simulink model "genericjosephtest"  (Simulink 10.3)
settings: Solver=ode45  StartTime=0.0  StopTime=inf  RelTol=1e-3  EnableMultiTasking=on
values from neighbouring files (symbols this model uses):
  ku = (Lr*m)/(Cyf*(Lf+Lr)) - (Lf*m)/(Cyr*(Lf+Lr))    (= -0.00270204285714)    [makePlants.m]
  Lf = 0.918    [makeBikeModel.m]    (also in makePlants.m)
  Lr = 0.612    [makeBikeModel.m]    (also in makePlants.m)
undefined symbols (not defined in the file or in its folder): Gains
libraries: CarMaker4SL x24, slctrlblks x2, pid_lib x2, simulink x1
(part 3 of 3)

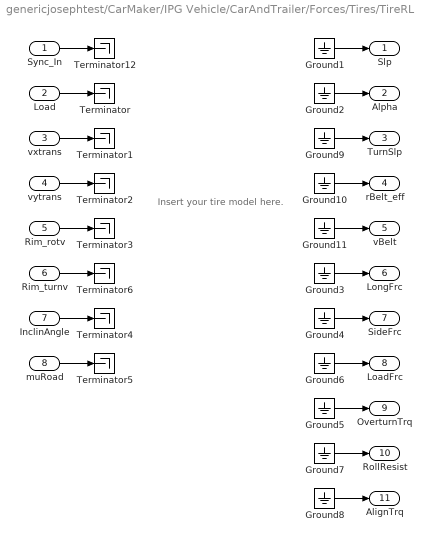
== system genericjosephtest/CarMaker/IPG Vehicle/CarAndTrailer/Forces/Tires/TireRL ==
  note: Insert your tire model here.
  Sync_In : Inport
  Load : Inport  Port=2
  vxtrans : Inport  Port=3
  vytrans : Inport  Port=4
  Rim_rotv : Inport  Port=5
  Rim_turnv : Inport  Port=6
  InclinAngle : Inport  Port=7
  muRoad : Inport  Port=8
  Ground{1..11} (11 alike) : Ground
  Terminator{,1..6,12} (8 alike) : Terminator
  Slp : Outport  VectorParamsAs1DForOutWhenUnconnected=off
  Alpha : Outport  Port=2  VectorParamsAs1DForOutWhenUnconnected=off
  TurnSlp : Outport  Port=3  VectorParamsAs1DForOutWhenUnconnected=off
  rBelt_eff : Outport  Port=4  VectorParamsAs1DForOutWhenUnconnected=off
  vBelt : Outport  Port=5  VectorParamsAs1DForOutWhenUnconnected=off
  LongFrc : Outport  Port=6  VectorParamsAs1DForOutWhenUnconnected=off
  SideFrc : Outport  Port=7  VectorParamsAs1DForOutWhenUnconnected=off
  LoadFrc : Outport  Port=8  VectorParamsAs1DForOutWhenUnconnected=off
  OverturnTrq : Outport  Port=9  VectorParamsAs1DForOutWhenUnconnected=off
  RollResist : Outport  Port=10  VectorParamsAs1DForOutWhenUnconnected=off
  AlignTrq : Outport  Port=11  VectorParamsAs1DForOutWhenUnconnected=off
  wires:
  Ground11/1 -> vBelt/1
  Ground10/1 -> rBelt_eff/1
  Ground9/1 -> TurnSlp/1
  Rim_turnv/1 -> Terminator6/1
  Sync_In/1 -> Terminator12/1
  Ground2/1 -> Alpha/1
  Ground3/1 -> LongFrc/1
  Ground4/1 -> SideFrc/1
  Ground5/1 -> OverturnTrq/1
  vxtrans/1 -> Terminator1/1
  vytrans/1 -> Terminator2/1
  Rim_rotv/1 -> Terminator3/1
  InclinAngle/1 -> Terminator4/1
  muRoad/1 -> Terminator5/1
  Load/1 -> Terminator/1
  Ground1/1 -> Slp/1
  Ground6/1 -> LoadFrc/1
  Ground7/1 -> RollResist/1
  Ground8/1 -> AlignTrq/1

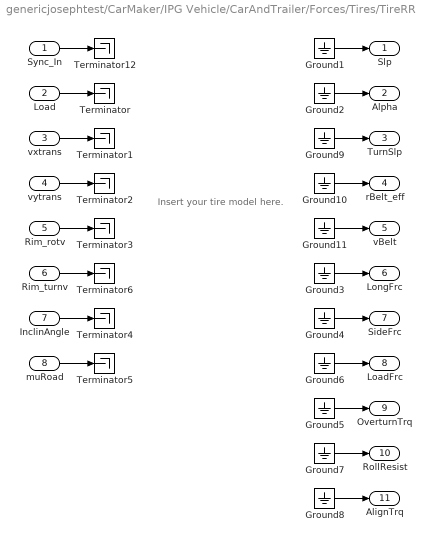
== system genericjosephtest/CarMaker/IPG Vehicle/CarAndTrailer/Forces/Tires/TireRR ==
  note: Insert your tire model here.
  Sync_In : Inport
  Load : Inport  Port=2
  vxtrans : Inport  Port=3
  vytrans : Inport  Port=4
  Rim_rotv : Inport  Port=5
  Rim_turnv : Inport  Port=6
  InclinAngle : Inport  Port=7
  muRoad : Inport  Port=8
  Ground{1..11} (11 alike) : Ground
  Terminator{,1..6,12} (8 alike) : Terminator
  Slp : Outport  VectorParamsAs1DForOutWhenUnconnected=off
  Alpha : Outport  Port=2  VectorParamsAs1DForOutWhenUnconnected=off
  TurnSlp : Outport  Port=3  VectorParamsAs1DForOutWhenUnconnected=off
  rBelt_eff : Outport  Port=4  VectorParamsAs1DForOutWhenUnconnected=off
  vBelt : Outport  Port=5  VectorParamsAs1DForOutWhenUnconnected=off
  LongFrc : Outport  Port=6  VectorParamsAs1DForOutWhenUnconnected=off
  SideFrc : Outport  Port=7  VectorParamsAs1DForOutWhenUnconnected=off
  LoadFrc : Outport  Port=8  VectorParamsAs1DForOutWhenUnconnected=off
  OverturnTrq : Outport  Port=9  VectorParamsAs1DForOutWhenUnconnected=off
  RollResist : Outport  Port=10  VectorParamsAs1DForOutWhenUnconnected=off
  AlignTrq : Outport  Port=11  VectorParamsAs1DForOutWhenUnconnected=off
  wires:
  Ground11/1 -> vBelt/1
  Ground10/1 -> rBelt_eff/1
  Ground9/1 -> TurnSlp/1
  Rim_turnv/1 -> Terminator6/1
  Sync_In/1 -> Terminator12/1
  Ground2/1 -> Alpha/1
  Ground3/1 -> LongFrc/1
  Ground4/1 -> SideFrc/1
  Ground5/1 -> OverturnTrq/1
  vxtrans/1 -> Terminator1/1
  vytrans/1 -> Terminator2/1
  Rim_rotv/1 -> Terminator3/1
  InclinAngle/1 -> Terminator4/1
  muRoad/1 -> Terminator5/1
  Load/1 -> Terminator/1
  Ground1/1 -> Slp/1
  Ground6/1 -> LoadFrc/1
  Ground7/1 -> RollResist/1
  Ground8/1 -> AlignTrq/1

== system genericjosephtest/CarMaker/IPG Vehicle/PowerTrain/MyPowerTrainXWD/Subsystem/Desired Yaw Rate Generator ==
  Linear Car Velocity : Inport
  steering angle : Inport  Port=2
  Add : Sum  Inputs=+++
  Constant : Constant  Value=0.8
  Constant1 : Constant  Value=ku
  Constant2 : Constant  Value=1.0
  Divide : Product  Inputs=*/
  Multiply : Product
  Multiply1 : Product
  Square : Math  Operator=square  SignedPower=on  SaturateOnIntegerOverflow=on
  Desired Yaw Rate : Outport  VectorParamsAs1DForOutWhenUnconnected=off
  wires:
  Constant1/1 -> Multiply/1
  steering angle/1 -> Multiply1/2
  Divide/1 -> Desired Yaw Rate/1
  Linear Car Velocity/1 -> Square/1, Multiply1/1
  Multiply/1 -> Add/1
  Multiply1/1 -> Divide/1
  Square/1 -> Multiply/2
  Constant/1 -> Add/2  "Lf - Distance between CG and front axel"
  Constant2/1 -> Add/3  "Lr - Distance between CG and rear axel"
  Add/1 -> Divide/2

== system genericjosephtest/CarMaker/IPG Vehicle/PowerTrain/MyPowerTrainXWD/Subsystem/Reference Yaw Rate Limiter ==
  note: Bind the reference yaw rate to the max possible yaw rate if the desired yaw rate is more than the max yaw rate possible
  note: Max Yaw Rate = tunability*mu*g/Vcg
  Vehicle Velocity : Inport
  Desired Yaw Rate : Inport  Port=2
  Add : Sum
  Constant : Constant  Value=2
  Constant1 : Constant  Value=0
  Divide : Product  Inputs=*/
  Divide1 : Product  Inputs=*/
  MATLAB Function : MATLAB Function  TreatAsAtomicUnit=on
  Multiply : Product
  Multiply1 : Product
  Read CM Dict : CarMaker4SL/Read CM Dict  xname=Car.muRoadRL  xsync=off
  Read CM Dict1 : CarMaker4SL/Read CM Dict  xname=Car.muRoadRR  xsync=off
  Saturation : Saturate  UpperLimit=10  LowerLimit=-10
  Switch : Switch  Criteria=u2 > Threshold  Threshold=1
  Tunability Factor : Constant
  g : Constant  Value=9.81
  Reference Yaw Rate : Outport  VectorParamsAs1DForOutWhenUnconnected=off
  wires:
  Desired Yaw Rate/1 -> Saturation/1
  MATLAB Function/1(ref_yaw) -> Reference Yaw Rate/1  "Reference Yaw Rate"
  Read CM Dict1/1 -> Add/2
  Read CM Dict/1 -> Add/1
  Add/1 -> Divide/1
  Constant/1 -> Divide/2
  Divide/1 -> Multiply/1  "mu (avg)"
  Multiply/1 -> Divide1/1
  Vehicle Velocity/1 -> Switch/2, Divide1/2
  g/1 -> Multiply/2
  Tunability Factor/1 -> Multiply1/2
  Multiply1/1 -> MATLAB Function/1(max_yaw)  "Max Yaw Rate"
  Divide1/1 -> Switch/1
  Constant1/1 -> Switch/3
  Switch/1 -> Multiply1/1
  Saturation/1 -> MATLAB Function/2(des_yaw)

== system genericjosephtest/CarMaker/IPG Vehicle/PowerTrain/MyPowerTrainXWD/Subsystem/Update PID Gains ==
  In1 : Inport
  Trigger : TriggerPort  TriggerType=falling  VariantControl=Variant  PortDimensions=1
  Bus Selector : BusSelector  OutputSignals=P,I,D,N
  Mux : Mux
  Write PID Gains : DataStoreWrite  DataStoreName=Gains  DataStoreElements=Gains(:)  IndexOptions=Index vector (dialog)  Indices=1  OutputSizes=1
  wires:
  Mux/1 -> Write PID Gains/1
  Bus Selector/2 -> Mux/2  "<I>"
  Bus Selector/1 -> Mux/1  "<P>"
  In1/1 -> Bus Selector/1
  Bus Selector/3 -> Mux/3  "<D>"
  Bus Selector/4 -> Mux/4  "<N>"

== matlab function CarMaker/IPG Vehicle/PowerTrain/MyPowerTrainXWD/Torque Distribution/Delta Torque Splitter ==
  data: steer_ang input double; moment_direction input double; Trq_RL output double; half_delta_Trq input double; Trq_RR output double
function [Trq_RL,Trq_RR] = split_delta_Trq(steer_ang, moment_direction,half_delta_Trq)
if abs(steer_ang) > 0.01    
    if moment_direction == 1
    %if desired yaw rate = positive (aka a left turn)
    %then need to subtract half delta torque to Rear Left, add to Rear Right
        Trq_RL = -half_delta_Trq;
        Trq_RR = half_delta_Trq;
    elseif moment_direction == -1
    %if desired yaw rate = negative (aka a right turn)
    %then need to add half delta torque to Rear Left, subtract from Rear Right
        Trq_RL = half_delta_Trq;
        Trq_RR = -half_delta_Trq;
    else
    %safety condition, add positve to both wheels
        Trq_RL = half_delta_Trq;
        Trq_RR = half_delta_Trq;
    end
else
   Trq_RL = 0;
   Trq_RR = 0; 
end

== matlab function CarMaker/IPG Vehicle/PowerTrain/MyPowerTrainXWD/Subsystem/Reference Yaw Rate Limiter/MATLAB Function ==
  data: max_yaw input double; ref_yaw output double; des_yaw input double
function ref_yaw = fcn(max_yaw, des_yaw)
    if abs(des_yaw) > max_yaw
        if des_yaw >= 0
            ref_yaw = max_yaw;
        else
            ref_yaw = -max_yaw;
        end      
    else 
        ref_yaw = des_yaw;
    end

== matlab function CarMaker/IPG Vehicle/PowerTrain/MyPowerTrainXWD/Reference Yaw Rate Limiter/MATLAB Function ==
  data: max_yaw input double; ref_yaw output double; des_yaw input double
function ref_yaw = fcn(max_yaw, des_yaw)
    if abs(des_yaw) > max_yaw
        if des_yaw >= 0
            ref_yaw = max_yaw;
        else
            ref_yaw = -max_yaw;
        end      
    else 
        ref_yaw = des_yaw;
    end
